simulink model "WSC_2023_Final_PVArray_Diode_All_Strings"  (R2023a)
settings: Solver=VariableStepAuto  StartTime=0.0  StopTime=1  FixedStep=Ts_Power  MinStep=0.0025  RelTol=1e-4
PreLoadFcn:
  | Ts_Power=5e-4;
  | Slope_Vdc=1;
InitFcn:
  | Ts_Power=50e-6;
  | Tc=1e-5;%break algebraic loop time constant
StopFcn:
  | if exist('I','var') && exist('V','var')
  |    figure(1)
  |    clf
  |    n=find(I>=0);
  |    n=n(end);
  |    Vglobal=V(1:n);
  |    Iglobal=I(1:n);
  | 
  | 
  |    Pglobal=Vglobal.*Iglobal;
  |    n=find(Pglobal==max(Pglobal));
  |    Pmax=Pglobal(n);
  |    Vmp=Vglobal(n);
  |    Imp=Iglobal(n);
  | 
  | 
  |    subplot(211)
  |    plot(Vglobal, Iglobal,Vmp,Imp,'or')
  |    ylabel('Current (A)')
  |    title(sprintf('Global I-V & P-V characteristics\n %s' ,ModuleName))
  | 
  | 
  |    subplot(212)
  |    plot(Vglobal, Pglobal,Vmp,Pmax,'or')
  |    ylabel('Power (W)')
  |    xlabel('Voltage (V)')
  | end
model workspace (MAT data in the model file):
  slope_Vdc = 3.0848387096
undefined symbols (not defined in the file or in its folder): Slope_Vdc_string1, Slope_Vdc_string2, Slope_Vdc_string3
libraries: spsPVArrayLib x257, spsVariableResistorLib x257, spsDiodeLib x55, spsCurrentMeasurementLib x3, spsVoltageMeasurementLib x3, spsControlledVoltageSourceLib x3, simulink x3, spspowerguiLib x3
(part 10 of 13)

== system WSC_2023_Final_PVArray_Diode_All_Strings/Subsystem22/PV7 ==
  Irr : Inport
  1PΩ : Constant  Value=1e15
  PV2 : spsPVArrayLib/PV Array  Npar=1  Nser=1  PlotType=array @ 25 deg.C & specified irradiances  S_vec="[ 1000  500  100 ]"  Temp_C_vec="[ 45 25  ]"  ModuleName=User-defined  PlotWhenSelected=off  Pm=3.8061  Ncell=1  Voc=0.7315  Isc=6.41  Vm=0.626  Im=6.08  beta_Voc_pc=-0.2256195755  alpha_Isc_pc=0.04692556634  beta_Voc=-0.0016504  alpha_Isc=0.0030079  IL=6.4137  I0=6.5578e-13  nI=0.95237  Rsh=7.312  Rs=0.0042689  RobustModel=on  RobustCellTemperature=25  BAL=on  Tc=1e-5  Tfilter=5e-5
  Terminator1 : Terminator
  Variable Resistor2 : spsVariableResistorLib/Variable Resistor  Rabsmin=1e-3
      settings: LibrarySourceBlock=sps_lib/Passives/Variable Resistor
  + : PMIOPort  Side=Left
  - : PMIOPort  Port=2  Side=Right
  wires:
  Irr/1 -> PV2/1
  1PΩ/1 -> Variable Resistor2/1
  PV2/1 -> Terminator1/1
  connections:
  -/RConn1 -- Variable Resistor2/RConn1 -- PV2/RConn2
  +/RConn1 -- Variable Resistor2/LConn1 -- PV2/RConn1

== system WSC_2023_Final_PVArray_Diode_All_Strings/Subsystem23/PV1 ==
  Irr : Inport
  1PΩ : Constant  Value=1e15
  PV2 : spsPVArrayLib/PV Array  Npar=1  Nser=1  PlotType=array @ 25 deg.C & specified irradiances  S_vec="[ 1000  500  100 ]"  Temp_C_vec="[ 45 25  ]"  ModuleName=User-defined  PlotWhenSelected=off  Pm=3.8061  Ncell=1  Voc=0.7315  Isc=6.41  Vm=0.626  Im=6.08  beta_Voc_pc=-0.2256195755  alpha_Isc_pc=0.04692556634  beta_Voc=-0.0016504  alpha_Isc=0.0030079  IL=6.4137  I0=6.5578e-13  nI=0.95237  Rsh=7.312  Rs=0.0042689  RobustModel=on  RobustCellTemperature=25  BAL=on  Tc=1e-5  Tfilter=5e-5
  Terminator1 : Terminator
  Variable Resistor2 : spsVariableResistorLib/Variable Resistor  Rabsmin=1e-3
      settings: LibrarySourceBlock=sps_lib/Passives/Variable Resistor
  + : PMIOPort  Side=Left
  - : PMIOPort  Port=2  Side=Right
  wires:
  Irr/1 -> PV2/1
  1PΩ/1 -> Variable Resistor2/1
  PV2/1 -> Terminator1/1
  connections:
  -/RConn1 -- Variable Resistor2/RConn1 -- PV2/RConn2
  +/RConn1 -- Variable Resistor2/LConn1 -- PV2/RConn1

== system WSC_2023_Final_PVArray_Diode_All_Strings/Subsystem23/PV2 ==
  Irr : Inport
  1PΩ : Constant  Value=1e15
  PV2 : spsPVArrayLib/PV Array  Npar=1  Nser=1  PlotType=array @ 25 deg.C & specified irradiances  S_vec="[ 1000  500  100 ]"  Temp_C_vec="[ 45 25  ]"  ModuleName=User-defined  PlotWhenSelected=off  Pm=3.8061  Ncell=1  Voc=0.7315  Isc=6.41  Vm=0.626  Im=6.08  beta_Voc_pc=-0.2256195755  alpha_Isc_pc=0.04692556634  beta_Voc=-0.0016504  alpha_Isc=0.0030079  IL=6.4137  I0=6.5578e-13  nI=0.95237  Rsh=7.312  Rs=0.0042689  RobustModel=on  RobustCellTemperature=25  BAL=on  Tc=1e-5  Tfilter=5e-5
  Terminator1 : Terminator
  Variable Resistor2 : spsVariableResistorLib/Variable Resistor  Rabsmin=1e-3
      settings: LibrarySourceBlock=sps_lib/Passives/Variable Resistor
  + : PMIOPort  Side=Left
  - : PMIOPort  Port=2  Side=Right
  wires:
  Irr/1 -> PV2/1
  1PΩ/1 -> Variable Resistor2/1
  PV2/1 -> Terminator1/1
  connections:
  -/RConn1 -- Variable Resistor2/RConn1 -- PV2/RConn2
  +/RConn1 -- Variable Resistor2/LConn1 -- PV2/RConn1

== system WSC_2023_Final_PVArray_Diode_All_Strings/Subsystem23/PV3 ==
  Irr : Inport
  1PΩ : Constant  Value=1e15
  PV2 : spsPVArrayLib/PV Array  Npar=1  Nser=1  PlotType=array @ 25 deg.C & specified irradiances  S_vec="[ 1000  500  100 ]"  Temp_C_vec="[ 45 25  ]"  ModuleName=User-defined  PlotWhenSelected=off  Pm=3.8061  Ncell=1  Voc=0.7315  Isc=6.41  Vm=0.626  Im=6.08  beta_Voc_pc=-0.2256195755  alpha_Isc_pc=0.04692556634  beta_Voc=-0.0016504  alpha_Isc=0.0030079  IL=6.4137  I0=6.5578e-13  nI=0.95237  Rsh=7.312  Rs=0.0042689  RobustModel=on  RobustCellTemperature=25  BAL=on  Tc=1e-5  Tfilter=5e-5
  Terminator1 : Terminator
  Variable Resistor2 : spsVariableResistorLib/Variable Resistor  Rabsmin=1e-3
      settings: LibrarySourceBlock=sps_lib/Passives/Variable Resistor
  + : PMIOPort  Side=Left
  - : PMIOPort  Port=2  Side=Right
  wires:
  Irr/1 -> PV2/1
  1PΩ/1 -> Variable Resistor2/1
  PV2/1 -> Terminator1/1
  connections:
  -/RConn1 -- Variable Resistor2/RConn1 -- PV2/RConn2
  +/RConn1 -- Variable Resistor2/LConn1 -- PV2/RConn1

== system WSC_2023_Final_PVArray_Diode_All_Strings/Subsystem23/PV4 ==
  Irr : Inport
  1PΩ : Constant  Value=1e15
  PV2 : spsPVArrayLib/PV Array  Npar=1  Nser=1  PlotType=array @ 25 deg.C & specified irradiances  S_vec="[ 1000  500  100 ]"  Temp_C_vec="[ 45 25  ]"  ModuleName=User-defined  PlotWhenSelected=off  Pm=3.8061  Ncell=1  Voc=0.7315  Isc=6.41  Vm=0.626  Im=6.08  beta_Voc_pc=-0.2256195755  alpha_Isc_pc=0.04692556634  beta_Voc=-0.0016504  alpha_Isc=0.0030079  IL=6.4137  I0=6.5578e-13  nI=0.95237  Rsh=7.312  Rs=0.0042689  RobustModel=on  RobustCellTemperature=25  BAL=on  Tc=1e-5  Tfilter=5e-5
  Terminator1 : Terminator
  Variable Resistor2 : spsVariableResistorLib/Variable Resistor  Rabsmin=1e-3
      settings: LibrarySourceBlock=sps_lib/Passives/Variable Resistor
  + : PMIOPort  Side=Left
  - : PMIOPort  Port=2  Side=Right
  wires:
  Irr/1 -> PV2/1
  1PΩ/1 -> Variable Resistor2/1
  PV2/1 -> Terminator1/1
  connections:
  -/RConn1 -- Variable Resistor2/RConn1 -- PV2/RConn2
  +/RConn1 -- Variable Resistor2/LConn1 -- PV2/RConn1

== system WSC_2023_Final_PVArray_Diode_All_Strings/Subsystem23/PV5 ==
  Irr : Inport
  1PΩ : Constant  Value=1e15
  PV2 : spsPVArrayLib/PV Array  Npar=1  Nser=1  PlotType=array @ 25 deg.C & specified irradiances  S_vec="[ 1000  500  100 ]"  Temp_C_vec="[ 45 25  ]"  ModuleName=User-defined  PlotWhenSelected=off  Pm=3.8061  Ncell=1  Voc=0.7315  Isc=6.41  Vm=0.626  Im=6.08  beta_Voc_pc=-0.2256195755  alpha_Isc_pc=0.04692556634  beta_Voc=-0.0016504  alpha_Isc=0.0030079  IL=6.4137  I0=6.5578e-13  nI=0.95237  Rsh=7.312  Rs=0.0042689  RobustModel=on  RobustCellTemperature=25  BAL=on  Tc=1e-5  Tfilter=5e-5
  Terminator1 : Terminator
  Variable Resistor2 : spsVariableResistorLib/Variable Resistor  Rabsmin=1e-3
      settings: LibrarySourceBlock=sps_lib/Passives/Variable Resistor
  + : PMIOPort  Side=Left
  - : PMIOPort  Port=2  Side=Right
  wires:
  Irr/1 -> PV2/1
  1PΩ/1 -> Variable Resistor2/1
  PV2/1 -> Terminator1/1
  connections:
  -/RConn1 -- Variable Resistor2/RConn1 -- PV2/RConn2
  +/RConn1 -- Variable Resistor2/LConn1 -- PV2/RConn1

== system WSC_2023_Final_PVArray_Diode_All_Strings/Subsystem23/PV6 ==
  Irr : Inport
  1PΩ : Constant  Value=1e15
  PV2 : spsPVArrayLib/PV Array  Npar=1  Nser=1  PlotType=array @ 25 deg.C & specified irradiances  S_vec="[ 1000  500  100 ]"  Temp_C_vec="[ 45 25  ]"  ModuleName=User-defined  PlotWhenSelected=off  Pm=3.8061  Ncell=1  Voc=0.7315  Isc=6.41  Vm=0.626  Im=6.08  beta_Voc_pc=-0.2256195755  alpha_Isc_pc=0.04692556634  beta_Voc=-0.0016504  alpha_Isc=0.0030079  IL=6.4137  I0=6.5578e-13  nI=0.95237  Rsh=7.312  Rs=0.0042689  RobustModel=on  RobustCellTemperature=25  BAL=on  Tc=1e-5  Tfilter=5e-5
  Terminator1 : Terminator
  Variable Resistor2 : spsVariableResistorLib/Variable Resistor  Rabsmin=1e-3
      settings: LibrarySourceBlock=sps_lib/Passives/Variable Resistor
  + : PMIOPort  Side=Left
  - : PMIOPort  Port=2  Side=Right
  wires:
  Irr/1 -> PV2/1
  1PΩ/1 -> Variable Resistor2/1
  PV2/1 -> Terminator1/1
  connections:
  -/RConn1 -- Variable Resistor2/RConn1 -- PV2/RConn2
  +/RConn1 -- Variable Resistor2/LConn1 -- PV2/RConn1

== system WSC_2023_Final_PVArray_Diode_All_Strings/Subsystem23/PV7 ==
  Irr : Inport
  1PΩ : Constant  Value=1e15
  PV2 : spsPVArrayLib/PV Array  Npar=1  Nser=1  PlotType=array @ 25 deg.C & specified irradiances  S_vec="[ 1000  500  100 ]"  Temp_C_vec="[ 45 25  ]"  ModuleName=User-defined  PlotWhenSelected=off  Pm=3.8061  Ncell=1  Voc=0.7315  Isc=6.41  Vm=0.626  Im=6.08  beta_Voc_pc=-0.2256195755  alpha_Isc_pc=0.04692556634  beta_Voc=-0.0016504  alpha_Isc=0.0030079  IL=6.4137  I0=6.5578e-13  nI=0.95237  Rsh=7.312  Rs=0.0042689  RobustModel=on  RobustCellTemperature=25  BAL=on  Tc=1e-5  Tfilter=5e-5
  Terminator1 : Terminator
  Variable Resistor2 : spsVariableResistorLib/Variable Resistor  Rabsmin=1e-3
      settings: LibrarySourceBlock=sps_lib/Passives/Variable Resistor
  + : PMIOPort  Side=Left
  - : PMIOPort  Port=2  Side=Right
  wires:
  Irr/1 -> PV2/1
  1PΩ/1 -> Variable Resistor2/1
  PV2/1 -> Terminator1/1
  connections:
  -/RConn1 -- Variable Resistor2/RConn1 -- PV2/RConn2
  +/RConn1 -- Variable Resistor2/LConn1 -- PV2/RConn1

== system WSC_2023_Final_PVArray_Diode_All_Strings/Subsystem24/PV1 ==
  Irr : Inport
  1PΩ : Constant  Value=1e15
  PV2 : spsPVArrayLib/PV Array  Npar=1  Nser=1  PlotType=array @ 25 deg.C & specified irradiances  S_vec="[ 1000  500  100 ]"  Temp_C_vec="[ 45 25  ]"  ModuleName=User-defined  PlotWhenSelected=off  Pm=3.8061  Ncell=1  Voc=0.7315  Isc=6.41  Vm=0.626  Im=6.08  beta_Voc_pc=-0.2256195755  alpha_Isc_pc=0.04692556634  beta_Voc=-0.0016504  alpha_Isc=0.0030079  IL=6.4137  I0=6.5578e-13  nI=0.95237  Rsh=7.312  Rs=0.0042689  RobustModel=on  RobustCellTemperature=25  BAL=on  Tc=1e-5  Tfilter=5e-5
  Terminator1 : Terminator
  Variable Resistor2 : spsVariableResistorLib/Variable Resistor  Rabsmin=1e-3
      settings: LibrarySourceBlock=sps_lib/Passives/Variable Resistor
  + : PMIOPort  Side=Left
  - : PMIOPort  Port=2  Side=Right
  wires:
  Irr/1 -> PV2/1
  1PΩ/1 -> Variable Resistor2/1
  PV2/1 -> Terminator1/1
  connections:
  -/RConn1 -- Variable Resistor2/RConn1 -- PV2/RConn2
  +/RConn1 -- Variable Resistor2/LConn1 -- PV2/RConn1

== system WSC_2023_Final_PVArray_Diode_All_Strings/Subsystem24/PV2 ==
  Irr : Inport
  1PΩ : Constant  Value=1e15
  PV2 : spsPVArrayLib/PV Array  Npar=1  Nser=1  PlotType=array @ 25 deg.C & specified irradiances  S_vec="[ 1000  500  100 ]"  Temp_C_vec="[ 45 25  ]"  ModuleName=User-defined  PlotWhenSelected=off  Pm=3.8061  Ncell=1  Voc=0.7315  Isc=6.41  Vm=0.626  Im=6.08  beta_Voc_pc=-0.2256195755  alpha_Isc_pc=0.04692556634  beta_Voc=-0.0016504  alpha_Isc=0.0030079  IL=6.4137  I0=6.5578e-13  nI=0.95237  Rsh=7.312  Rs=0.0042689  RobustModel=on  RobustCellTemperature=25  BAL=on  Tc=1e-5  Tfilter=5e-5
  Terminator1 : Terminator
  Variable Resistor2 : spsVariableResistorLib/Variable Resistor  Rabsmin=1e-3
      settings: LibrarySourceBlock=sps_lib/Passives/Variable Resistor
  + : PMIOPort  Side=Left
  - : PMIOPort  Port=2  Side=Right
  wires:
  Irr/1 -> PV2/1
  1PΩ/1 -> Variable Resistor2/1
  PV2/1 -> Terminator1/1
  connections:
  -/RConn1 -- Variable Resistor2/RConn1 -- PV2/RConn2
  +/RConn1 -- Variable Resistor2/LConn1 -- PV2/RConn1

== system WSC_2023_Final_PVArray_Diode_All_Strings/Subsystem24/PV3 ==
  Irr : Inport
  1PΩ : Constant  Value=1e15
  PV2 : spsPVArrayLib/PV Array  Npar=1  Nser=1  PlotType=array @ 25 deg.C & specified irradiances  S_vec="[ 1000  500  100 ]"  Temp_C_vec="[ 45 25  ]"  ModuleName=User-defined  PlotWhenSelected=off  Pm=3.8061  Ncell=1  Voc=0.7315  Isc=6.41  Vm=0.626  Im=6.08  beta_Voc_pc=-0.2256195755  alpha_Isc_pc=0.04692556634  beta_Voc=-0.0016504  alpha_Isc=0.0030079  IL=6.4137  I0=6.5578e-13  nI=0.95237  Rsh=7.312  Rs=0.0042689  RobustModel=on  RobustCellTemperature=25  BAL=on  Tc=1e-5  Tfilter=5e-5
  Terminator1 : Terminator
  Variable Resistor2 : spsVariableResistorLib/Variable Resistor  Rabsmin=1e-3
      settings: LibrarySourceBlock=sps_lib/Passives/Variable Resistor
  + : PMIOPort  Side=Left
  - : PMIOPort  Port=2  Side=Right
  wires:
  Irr/1 -> PV2/1
  1PΩ/1 -> Variable Resistor2/1
  PV2/1 -> Terminator1/1
  connections:
  -/RConn1 -- Variable Resistor2/RConn1 -- PV2/RConn2
  +/RConn1 -- Variable Resistor2/LConn1 -- PV2/RConn1

== system WSC_2023_Final_PVArray_Diode_All_Strings/Subsystem24/PV4 ==
  Irr : Inport
  1PΩ : Constant  Value=1e15
  PV2 : spsPVArrayLib/PV Array  Npar=1  Nser=1  PlotType=array @ 25 deg.C & specified irradiances  S_vec="[ 1000  500  100 ]"  Temp_C_vec="[ 45 25  ]"  ModuleName=User-defined  PlotWhenSelected=off  Pm=3.8061  Ncell=1  Voc=0.7315  Isc=6.41  Vm=0.626  Im=6.08  beta_Voc_pc=-0.2256195755  alpha_Isc_pc=0.04692556634  beta_Voc=-0.0016504  alpha_Isc=0.0030079  IL=6.4137  I0=6.5578e-13  nI=0.95237  Rsh=7.312  Rs=0.0042689  RobustModel=on  RobustCellTemperature=25  BAL=on  Tc=1e-5  Tfilter=5e-5
  Terminator1 : Terminator
  Variable Resistor2 : spsVariableResistorLib/Variable Resistor  Rabsmin=1e-3
      settings: LibrarySourceBlock=sps_lib/Passives/Variable Resistor
  + : PMIOPort  Side=Left
  - : PMIOPort  Port=2  Side=Right
  wires:
  Irr/1 -> PV2/1
  1PΩ/1 -> Variable Resistor2/1
  PV2/1 -> Terminator1/1
  connections:
  -/RConn1 -- Variable Resistor2/RConn1 -- PV2/RConn2
  +/RConn1 -- Variable Resistor2/LConn1 -- PV2/RConn1

== system WSC_2023_Final_PVArray_Diode_All_Strings/Subsystem24/PV5 ==
  Irr : Inport
  1PΩ : Constant  Value=1e15
  PV2 : spsPVArrayLib/PV Array  Npar=1  Nser=1  PlotType=array @ 25 deg.C & specified irradiances  S_vec="[ 1000  500  100 ]"  Temp_C_vec="[ 45 25  ]"  ModuleName=User-defined  PlotWhenSelected=off  Pm=3.8061  Ncell=1  Voc=0.7315  Isc=6.41  Vm=0.626  Im=6.08  beta_Voc_pc=-0.2256195755  alpha_Isc_pc=0.04692556634  beta_Voc=-0.0016504  alpha_Isc=0.0030079  IL=6.4137  I0=6.5578e-13  nI=0.95237  Rsh=7.312  Rs=0.0042689  RobustModel=on  RobustCellTemperature=25  BAL=on  Tc=1e-5  Tfilter=5e-5
  Terminator1 : Terminator
  Variable Resistor2 : spsVariableResistorLib/Variable Resistor  Rabsmin=1e-3
      settings: LibrarySourceBlock=sps_lib/Passives/Variable Resistor
  + : PMIOPort  Side=Left
  - : PMIOPort  Port=2  Side=Right
  wires:
  Irr/1 -> PV2/1
  1PΩ/1 -> Variable Resistor2/1
  PV2/1 -> Terminator1/1
  connections:
  -/RConn1 -- Variable Resistor2/RConn1 -- PV2/RConn2
  +/RConn1 -- Variable Resistor2/LConn1 -- PV2/RConn1

== system WSC_2023_Final_PVArray_Diode_All_Strings/Subsystem24/PV6 ==
  Irr : Inport
  1PΩ : Constant  Value=1e15
  PV2 : spsPVArrayLib/PV Array  Npar=1  Nser=1  PlotType=array @ 25 deg.C & specified irradiances  S_vec="[ 1000  500  100 ]"  Temp_C_vec="[ 45 25  ]"  ModuleName=User-defined  PlotWhenSelected=off  Pm=3.8061  Ncell=1  Voc=0.7315  Isc=6.41  Vm=0.626  Im=6.08  beta_Voc_pc=-0.2256195755  alpha_Isc_pc=0.04692556634  beta_Voc=-0.0016504  alpha_Isc=0.0030079  IL=6.4137  I0=6.5578e-13  nI=0.95237  Rsh=7.312  Rs=0.0042689  RobustModel=on  RobustCellTemperature=25  BAL=on  Tc=1e-5  Tfilter=5e-5
  Terminator1 : Terminator
  Variable Resistor2 : spsVariableResistorLib/Variable Resistor  Rabsmin=1e-3
      settings: LibrarySourceBlock=sps_lib/Passives/Variable Resistor
  + : PMIOPort  Side=Left
  - : PMIOPort  Port=2  Side=Right
  wires:
  Irr/1 -> PV2/1
  1PΩ/1 -> Variable Resistor2/1
  PV2/1 -> Terminator1/1
  connections:
  -/RConn1 -- Variable Resistor2/RConn1 -- PV2/RConn2
  +/RConn1 -- Variable Resistor2/LConn1 -- PV2/RConn1

== system WSC_2023_Final_PVArray_Diode_All_Strings/Subsystem24/PV7 ==
  Irr : Inport
  1PΩ : Constant  Value=1e15
  PV2 : spsPVArrayLib/PV Array  Npar=1  Nser=1  PlotType=array @ 25 deg.C & specified irradiances  S_vec="[ 1000  500  100 ]"  Temp_C_vec="[ 45 25  ]"  ModuleName=User-defined  PlotWhenSelected=off  Pm=3.8061  Ncell=1  Voc=0.7315  Isc=6.41  Vm=0.626  Im=6.08  beta_Voc_pc=-0.2256195755  alpha_Isc_pc=0.04692556634  beta_Voc=-0.0016504  alpha_Isc=0.0030079  IL=6.4137  I0=6.5578e-13  nI=0.95237  Rsh=7.312  Rs=0.0042689  RobustModel=on  RobustCellTemperature=25  BAL=on  Tc=1e-5  Tfilter=5e-5
  Terminator1 : Terminator
  Variable Resistor2 : spsVariableResistorLib/Variable Resistor  Rabsmin=1e-3
      settings: LibrarySourceBlock=sps_lib/Passives/Variable Resistor
  + : PMIOPort  Side=Left
  - : PMIOPort  Port=2  Side=Right
  wires:
  Irr/1 -> PV2/1
  1PΩ/1 -> Variable Resistor2/1
  PV2/1 -> Terminator1/1
  connections:
  -/RConn1 -- Variable Resistor2/RConn1 -- PV2/RConn2
  +/RConn1 -- Variable Resistor2/LConn1 -- PV2/RConn1

== system WSC_2023_Final_PVArray_Diode_All_Strings/Subsystem26/PV1 ==
  Irr : Inport
  1PΩ : Constant  Value=1e15
  PV2 : spsPVArrayLib/PV Array  Npar=1  Nser=1  PlotType=array @ 25 deg.C & specified irradiances  S_vec="[ 1000  500  100 ]"  Temp_C_vec="[ 45 25  ]"  ModuleName=User-defined  PlotWhenSelected=off  Pm=3.8061  Ncell=1  Voc=0.7315  Isc=6.41  Vm=0.626  Im=6.08  beta_Voc_pc=-0.2256195755  alpha_Isc_pc=0.04692556634  beta_Voc=-0.0016504  alpha_Isc=0.0030079  IL=6.4137  I0=6.5578e-13  nI=0.95237  Rsh=7.312  Rs=0.0042689  RobustModel=on  RobustCellTemperature=25  BAL=on  Tc=1e-5  Tfilter=5e-5
  Terminator1 : Terminator
  Variable Resistor2 : spsVariableResistorLib/Variable Resistor  Rabsmin=1e-3
      settings: LibrarySourceBlock=sps_lib/Passives/Variable Resistor
  + : PMIOPort  Side=Left
  - : PMIOPort  Port=2  Side=Right
  wires:
  Irr/1 -> PV2/1
  1PΩ/1 -> Variable Resistor2/1
  PV2/1 -> Terminator1/1
  connections:
  -/RConn1 -- Variable Resistor2/RConn1 -- PV2/RConn2
  +/RConn1 -- Variable Resistor2/LConn1 -- PV2/RConn1

== system WSC_2023_Final_PVArray_Diode_All_Strings/Subsystem26/PV2 ==
  Irr : Inport
  1PΩ : Constant  Value=1e15
  PV2 : spsPVArrayLib/PV Array  Npar=1  Nser=1  PlotType=array @ 25 deg.C & specified irradiances  S_vec="[ 1000  500  100 ]"  Temp_C_vec="[ 45 25  ]"  ModuleName=User-defined  PlotWhenSelected=off  Pm=3.8061  Ncell=1  Voc=0.7315  Isc=6.41  Vm=0.626  Im=6.08  beta_Voc_pc=-0.2256195755  alpha_Isc_pc=0.04692556634  beta_Voc=-0.0016504  alpha_Isc=0.0030079  IL=6.4137  I0=6.5578e-13  nI=0.95237  Rsh=7.312  Rs=0.0042689  RobustModel=on  RobustCellTemperature=25  BAL=on  Tc=1e-5  Tfilter=5e-5
  Terminator1 : Terminator
  Variable Resistor2 : spsVariableResistorLib/Variable Resistor  Rabsmin=1e-3
      settings: LibrarySourceBlock=sps_lib/Passives/Variable Resistor
  + : PMIOPort  Side=Left
  - : PMIOPort  Port=2  Side=Right
  wires:
  Irr/1 -> PV2/1
  1PΩ/1 -> Variable Resistor2/1
  PV2/1 -> Terminator1/1
  connections:
  -/RConn1 -- Variable Resistor2/RConn1 -- PV2/RConn2
  +/RConn1 -- Variable Resistor2/LConn1 -- PV2/RConn1

== system WSC_2023_Final_PVArray_Diode_All_Strings/Subsystem26/PV3 ==
  Irr : Inport
  1PΩ : Constant  Value=1e15
  PV2 : spsPVArrayLib/PV Array  Npar=1  Nser=1  PlotType=array @ 25 deg.C & specified irradiances  S_vec="[ 1000  500  100 ]"  Temp_C_vec="[ 45 25  ]"  ModuleName=User-defined  PlotWhenSelected=off  Pm=3.8061  Ncell=1  Voc=0.7315  Isc=6.41  Vm=0.626  Im=6.08  beta_Voc_pc=-0.2256195755  alpha_Isc_pc=0.04692556634  beta_Voc=-0.0016504  alpha_Isc=0.0030079  IL=6.4137  I0=6.5578e-13  nI=0.95237  Rsh=7.312  Rs=0.0042689  RobustModel=on  RobustCellTemperature=25  BAL=on  Tc=1e-5  Tfilter=5e-5
  Terminator1 : Terminator
  Variable Resistor2 : spsVariableResistorLib/Variable Resistor  Rabsmin=1e-3
      settings: LibrarySourceBlock=sps_lib/Passives/Variable Resistor
  + : PMIOPort  Side=Left
  - : PMIOPort  Port=2  Side=Right
  wires:
  Irr/1 -> PV2/1
  1PΩ/1 -> Variable Resistor2/1
  PV2/1 -> Terminator1/1
  connections:
  -/RConn1 -- Variable Resistor2/RConn1 -- PV2/RConn2
  +/RConn1 -- Variable Resistor2/LConn1 -- PV2/RConn1

== system WSC_2023_Final_PVArray_Diode_All_Strings/Subsystem26/PV4 ==
  Irr : Inport
  1PΩ : Constant  Value=1e15
  PV2 : spsPVArrayLib/PV Array  Npar=1  Nser=1  PlotType=array @ 25 deg.C & specified irradiances  S_vec="[ 1000  500  100 ]"  Temp_C_vec="[ 45 25  ]"  ModuleName=User-defined  PlotWhenSelected=off  Pm=3.8061  Ncell=1  Voc=0.7315  Isc=6.41  Vm=0.626  Im=6.08  beta_Voc_pc=-0.2256195755  alpha_Isc_pc=0.04692556634  beta_Voc=-0.0016504  alpha_Isc=0.0030079  IL=6.4137  I0=6.5578e-13  nI=0.95237  Rsh=7.312  Rs=0.0042689  RobustModel=on  RobustCellTemperature=25  BAL=on  Tc=1e-5  Tfilter=5e-5
  Terminator1 : Terminator
  Variable Resistor2 : spsVariableResistorLib/Variable Resistor  Rabsmin=1e-3
      settings: LibrarySourceBlock=sps_lib/Passives/Variable Resistor
  + : PMIOPort  Side=Left
  - : PMIOPort  Port=2  Side=Right
  wires:
  Irr/1 -> PV2/1
  1PΩ/1 -> Variable Resistor2/1
  PV2/1 -> Terminator1/1
  connections:
  -/RConn1 -- Variable Resistor2/RConn1 -- PV2/RConn2
  +/RConn1 -- Variable Resistor2/LConn1 -- PV2/RConn1

== system WSC_2023_Final_PVArray_Diode_All_Strings/Subsystem26/PV5 ==
  Irr : Inport
  1PΩ : Constant  Value=1e15
  PV2 : spsPVArrayLib/PV Array  Npar=1  Nser=1  PlotType=array @ 25 deg.C & specified irradiances  S_vec="[ 1000  500  100 ]"  Temp_C_vec="[ 45 25  ]"  ModuleName=User-defined  PlotWhenSelected=off  Pm=3.8061  Ncell=1  Voc=0.7315  Isc=6.41  Vm=0.626  Im=6.08  beta_Voc_pc=-0.2256195755  alpha_Isc_pc=0.04692556634  beta_Voc=-0.0016504  alpha_Isc=0.0030079  IL=6.4137  I0=6.5578e-13  nI=0.95237  Rsh=7.312  Rs=0.0042689  RobustModel=on  RobustCellTemperature=25  BAL=on  Tc=1e-5  Tfilter=5e-5
  Terminator1 : Terminator
  Variable Resistor2 : spsVariableResistorLib/Variable Resistor  Rabsmin=1e-3
      settings: LibrarySourceBlock=sps_lib/Passives/Variable Resistor
  + : PMIOPort  Side=Left
  - : PMIOPort  Port=2  Side=Right
  wires:
  Irr/1 -> PV2/1
  1PΩ/1 -> Variable Resistor2/1
  PV2/1 -> Terminator1/1
  connections:
  -/RConn1 -- Variable Resistor2/RConn1 -- PV2/RConn2
  +/RConn1 -- Variable Resistor2/LConn1 -- PV2/RConn1

== system WSC_2023_Final_PVArray_Diode_All_Strings/Subsystem26/PV6 ==
  Irr : Inport
  1PΩ : Constant  Value=1e15
  PV2 : spsPVArrayLib/PV Array  Npar=1  Nser=1  PlotType=array @ 25 deg.C & specified irradiances  S_vec="[ 1000  500  100 ]"  Temp_C_vec="[ 45 25  ]"  ModuleName=User-defined  PlotWhenSelected=off  Pm=3.8061  Ncell=1  Voc=0.7315  Isc=6.41  Vm=0.626  Im=6.08  beta_Voc_pc=-0.2256195755  alpha_Isc_pc=0.04692556634  beta_Voc=-0.0016504  alpha_Isc=0.0030079  IL=6.4137  I0=6.5578e-13  nI=0.95237  Rsh=7.312  Rs=0.0042689  RobustModel=on  RobustCellTemperature=25  BAL=on  Tc=1e-5  Tfilter=5e-5
  Terminator1 : Terminator
  Variable Resistor2 : spsVariableResistorLib/Variable Resistor  Rabsmin=1e-3
      settings: LibrarySourceBlock=sps_lib/Passives/Variable Resistor
  + : PMIOPort  Side=Left
  - : PMIOPort  Port=2  Side=Right
  wires:
  Irr/1 -> PV2/1
  1PΩ/1 -> Variable Resistor2/1
  PV2/1 -> Terminator1/1
  connections:
  -/RConn1 -- Variable Resistor2/RConn1 -- PV2/RConn2
  +/RConn1 -- Variable Resistor2/LConn1 -- PV2/RConn1

== system WSC_2023_Final_PVArray_Diode_All_Strings/Subsystem27/PV1 ==
  Irr : Inport
  1PΩ : Constant  Value=1e15
  PV2 : spsPVArrayLib/PV Array  Npar=1  Nser=1  PlotType=array @ 25 deg.C & specified irradiances  S_vec="[ 1000  500  100 ]"  Temp_C_vec="[ 45 25  ]"  ModuleName=User-defined  PlotWhenSelected=off  Pm=3.8061  Ncell=1  Voc=0.7315  Isc=6.41  Vm=0.626  Im=6.08  beta_Voc_pc=-0.2256195755  alpha_Isc_pc=0.04692556634  beta_Voc=-0.0016504  alpha_Isc=0.0030079  IL=6.4137  I0=6.5578e-13  nI=0.95237  Rsh=7.312  Rs=0.0042689  RobustModel=on  RobustCellTemperature=25  BAL=on  Tc=1e-5  Tfilter=5e-5
  Terminator1 : Terminator
  Variable Resistor2 : spsVariableResistorLib/Variable Resistor  Rabsmin=1e-3
      settings: LibrarySourceBlock=sps_lib/Passives/Variable Resistor
  + : PMIOPort  Side=Left
  - : PMIOPort  Port=2  Side=Right
  wires:
  Irr/1 -> PV2/1
  1PΩ/1 -> Variable Resistor2/1
  PV2/1 -> Terminator1/1
  connections:
  -/RConn1 -- Variable Resistor2/RConn1 -- PV2/RConn2
  +/RConn1 -- Variable Resistor2/LConn1 -- PV2/RConn1

== system WSC_2023_Final_PVArray_Diode_All_Strings/Subsystem27/PV2 ==
  Irr : Inport
  1PΩ : Constant  Value=1e15
  PV2 : spsPVArrayLib/PV Array  Npar=1  Nser=1  PlotType=array @ 25 deg.C & specified irradiances  S_vec="[ 1000  500  100 ]"  Temp_C_vec="[ 45 25  ]"  ModuleName=User-defined  PlotWhenSelected=off  Pm=3.8061  Ncell=1  Voc=0.7315  Isc=6.41  Vm=0.626  Im=6.08  beta_Voc_pc=-0.2256195755  alpha_Isc_pc=0.04692556634  beta_Voc=-0.0016504  alpha_Isc=0.0030079  IL=6.4137  I0=6.5578e-13  nI=0.95237  Rsh=7.312  Rs=0.0042689  RobustModel=on  RobustCellTemperature=25  BAL=on  Tc=1e-5  Tfilter=5e-5
  Terminator1 : Terminator
  Variable Resistor2 : spsVariableResistorLib/Variable Resistor  Rabsmin=1e-3
      settings: LibrarySourceBlock=sps_lib/Passives/Variable Resistor
  + : PMIOPort  Side=Left
  - : PMIOPort  Port=2  Side=Right
  wires:
  Irr/1 -> PV2/1
  1PΩ/1 -> Variable Resistor2/1
  PV2/1 -> Terminator1/1
  connections:
  -/RConn1 -- Variable Resistor2/RConn1 -- PV2/RConn2
  +/RConn1 -- Variable Resistor2/LConn1 -- PV2/RConn1

== system WSC_2023_Final_PVArray_Diode_All_Strings/Subsystem27/PV3 ==
  Irr : Inport
  1PΩ : Constant  Value=1e15
  PV2 : spsPVArrayLib/PV Array  Npar=1  Nser=1  PlotType=array @ 25 deg.C & specified irradiances  S_vec="[ 1000  500  100 ]"  Temp_C_vec="[ 45 25  ]"  ModuleName=User-defined  PlotWhenSelected=off  Pm=3.8061  Ncell=1  Voc=0.7315  Isc=6.41  Vm=0.626  Im=6.08  beta_Voc_pc=-0.2256195755  alpha_Isc_pc=0.04692556634  beta_Voc=-0.0016504  alpha_Isc=0.0030079  IL=6.4137  I0=6.5578e-13  nI=0.95237  Rsh=7.312  Rs=0.0042689  RobustModel=on  RobustCellTemperature=25  BAL=on  Tc=1e-5  Tfilter=5e-5
  Terminator1 : Terminator
  Variable Resistor2 : spsVariableResistorLib/Variable Resistor  Rabsmin=1e-3
      settings: LibrarySourceBlock=sps_lib/Passives/Variable Resistor
  + : PMIOPort  Side=Left
  - : PMIOPort  Port=2  Side=Right
  wires:
  Irr/1 -> PV2/1
  1PΩ/1 -> Variable Resistor2/1
  PV2/1 -> Terminator1/1
  connections:
  -/RConn1 -- Variable Resistor2/RConn1 -- PV2/RConn2
  +/RConn1 -- Variable Resistor2/LConn1 -- PV2/RConn1

== system WSC_2023_Final_PVArray_Diode_All_Strings/Subsystem27/PV4 ==
  Irr : Inport
  1PΩ : Constant  Value=1e15
  PV2 : spsPVArrayLib/PV Array  Npar=1  Nser=1  PlotType=array @ 25 deg.C & specified irradiances  S_vec="[ 1000  500  100 ]"  Temp_C_vec="[ 45 25  ]"  ModuleName=User-defined  PlotWhenSelected=off  Pm=3.8061  Ncell=1  Voc=0.7315  Isc=6.41  Vm=0.626  Im=6.08  beta_Voc_pc=-0.2256195755  alpha_Isc_pc=0.04692556634  beta_Voc=-0.0016504  alpha_Isc=0.0030079  IL=6.4137  I0=6.5578e-13  nI=0.95237  Rsh=7.312  Rs=0.0042689  RobustModel=on  RobustCellTemperature=25  BAL=on  Tc=1e-5  Tfilter=5e-5
  Terminator1 : Terminator
  Variable Resistor2 : spsVariableResistorLib/Variable Resistor  Rabsmin=1e-3
      settings: LibrarySourceBlock=sps_lib/Passives/Variable Resistor
  + : PMIOPort  Side=Left
  - : PMIOPort  Port=2  Side=Right
  wires:
  Irr/1 -> PV2/1
  1PΩ/1 -> Variable Resistor2/1
  PV2/1 -> Terminator1/1
  connections:
  -/RConn1 -- Variable Resistor2/RConn1 -- PV2/RConn2
  +/RConn1 -- Variable Resistor2/LConn1 -- PV2/RConn1

== system WSC_2023_Final_PVArray_Diode_All_Strings/Subsystem27/PV5 ==
  Irr : Inport
  1PΩ : Constant  Value=1e15
  PV2 : spsPVArrayLib/PV Array  Npar=1  Nser=1  PlotType=array @ 25 deg.C & specified irradiances  S_vec="[ 1000  500  100 ]"  Temp_C_vec="[ 45 25  ]"  ModuleName=User-defined  PlotWhenSelected=off  Pm=3.8061  Ncell=1  Voc=0.7315  Isc=6.41  Vm=0.626  Im=6.08  beta_Voc_pc=-0.2256195755  alpha_Isc_pc=0.04692556634  beta_Voc=-0.0016504  alpha_Isc=0.0030079  IL=6.4137  I0=6.5578e-13  nI=0.95237  Rsh=7.312  Rs=0.0042689  RobustModel=on  RobustCellTemperature=25  BAL=on  Tc=1e-5  Tfilter=5e-5
  Terminator1 : Terminator
  Variable Resistor2 : spsVariableResistorLib/Variable Resistor  Rabsmin=1e-3
      settings: LibrarySourceBlock=sps_lib/Passives/Variable Resistor
  + : PMIOPort  Side=Left
  - : PMIOPort  Port=2  Side=Right
  wires:
  Irr/1 -> PV2/1
  1PΩ/1 -> Variable Resistor2/1
  PV2/1 -> Terminator1/1
  connections:
  -/RConn1 -- Variable Resistor2/RConn1 -- PV2/RConn2
  +/RConn1 -- Variable Resistor2/LConn1 -- PV2/RConn1

== system WSC_2023_Final_PVArray_Diode_All_Strings/Subsystem27/PV6 ==
  Irr : Inport
  1PΩ : Constant  Value=1e15
  PV2 : spsPVArrayLib/PV Array  Npar=1  Nser=1  PlotType=array @ 25 deg.C & specified irradiances  S_vec="[ 1000  500  100 ]"  Temp_C_vec="[ 45 25  ]"  ModuleName=User-defined  PlotWhenSelected=off  Pm=3.8061  Ncell=1  Voc=0.7315  Isc=6.41  Vm=0.626  Im=6.08  beta_Voc_pc=-0.2256195755  alpha_Isc_pc=0.04692556634  beta_Voc=-0.0016504  alpha_Isc=0.0030079  IL=6.4137  I0=6.5578e-13  nI=0.95237  Rsh=7.312  Rs=0.0042689  RobustModel=on  RobustCellTemperature=25  BAL=on  Tc=1e-5  Tfilter=5e-5
  Terminator1 : Terminator
  Variable Resistor2 : spsVariableResistorLib/Variable Resistor  Rabsmin=1e-3
      settings: LibrarySourceBlock=sps_lib/Passives/Variable Resistor
  + : PMIOPort  Side=Left
  - : PMIOPort  Port=2  Side=Right
  wires:
  Irr/1 -> PV2/1
  1PΩ/1 -> Variable Resistor2/1
  PV2/1 -> Terminator1/1
  connections:
  -/RConn1 -- Variable Resistor2/RConn1 -- PV2/RConn2
  +/RConn1 -- Variable Resistor2/LConn1 -- PV2/RConn1

== system WSC_2023_Final_PVArray_Diode_All_Strings/Subsystem28/PV1 ==
  Irr : Inport
  1PΩ : Constant  Value=1e15
  PV2 : spsPVArrayLib/PV Array  Npar=1  Nser=1  PlotType=array @ 25 deg.C & specified irradiances  S_vec="[ 1000  500  100 ]"  Temp_C_vec="[ 45 25  ]"  ModuleName=User-defined  PlotWhenSelected=off  Pm=3.8061  Ncell=1  Voc=0.7315  Isc=6.41  Vm=0.626  Im=6.08  beta_Voc_pc=-0.2256195755  alpha_Isc_pc=0.04692556634  beta_Voc=-0.0016504  alpha_Isc=0.0030079  IL=6.4137  I0=6.5578e-13  nI=0.95237  Rsh=7.312  Rs=0.0042689  RobustModel=on  RobustCellTemperature=25  BAL=on  Tc=1e-5  Tfilter=5e-5
  Terminator1 : Terminator
  Variable Resistor2 : spsVariableResistorLib/Variable Resistor  Rabsmin=1e-3
      settings: LibrarySourceBlock=sps_lib/Passives/Variable Resistor
  + : PMIOPort  Side=Left
  - : PMIOPort  Port=2  Side=Right
  wires:
  Irr/1 -> PV2/1
  1PΩ/1 -> Variable Resistor2/1
  PV2/1 -> Terminator1/1
  connections:
  -/RConn1 -- Variable Resistor2/RConn1 -- PV2/RConn2
  +/RConn1 -- Variable Resistor2/LConn1 -- PV2/RConn1

== system WSC_2023_Final_PVArray_Diode_All_Strings/Subsystem28/PV2 ==
  Irr : Inport
  1PΩ : Constant  Value=1e15
  PV2 : spsPVArrayLib/PV Array  Npar=1  Nser=1  PlotType=array @ 25 deg.C & specified irradiances  S_vec="[ 1000  500  100 ]"  Temp_C_vec="[ 45 25  ]"  ModuleName=User-defined  PlotWhenSelected=off  Pm=3.8061  Ncell=1  Voc=0.7315  Isc=6.41  Vm=0.626  Im=6.08  beta_Voc_pc=-0.2256195755  alpha_Isc_pc=0.04692556634  beta_Voc=-0.0016504  alpha_Isc=0.0030079  IL=6.4137  I0=6.5578e-13  nI=0.95237  Rsh=7.312  Rs=0.0042689  RobustModel=on  RobustCellTemperature=25  BAL=on  Tc=1e-5  Tfilter=5e-5
  Terminator1 : Terminator
  Variable Resistor2 : spsVariableResistorLib/Variable Resistor  Rabsmin=1e-3
      settings: LibrarySourceBlock=sps_lib/Passives/Variable Resistor
  + : PMIOPort  Side=Left
  - : PMIOPort  Port=2  Side=Right
  wires:
  Irr/1 -> PV2/1
  1PΩ/1 -> Variable Resistor2/1
  PV2/1 -> Terminator1/1
  connections:
  -/RConn1 -- Variable Resistor2/RConn1 -- PV2/RConn2
  +/RConn1 -- Variable Resistor2/LConn1 -- PV2/RConn1

== system WSC_2023_Final_PVArray_Diode_All_Strings/Subsystem28/PV3 ==
  Irr : Inport
  1PΩ : Constant  Value=1e15
  PV2 : spsPVArrayLib/PV Array  Npar=1  Nser=1  PlotType=array @ 25 deg.C & specified irradiances  S_vec="[ 1000  500  100 ]"  Temp_C_vec="[ 45 25  ]"  ModuleName=User-defined  PlotWhenSelected=off  Pm=3.8061  Ncell=1  Voc=0.7315  Isc=6.41  Vm=0.626  Im=6.08  beta_Voc_pc=-0.2256195755  alpha_Isc_pc=0.04692556634  beta_Voc=-0.0016504  alpha_Isc=0.0030079  IL=6.4137  I0=6.5578e-13  nI=0.95237  Rsh=7.312  Rs=0.0042689  RobustModel=on  RobustCellTemperature=25  BAL=on  Tc=1e-5  Tfilter=5e-5
  Terminator1 : Terminator
  Variable Resistor2 : spsVariableResistorLib/Variable Resistor  Rabsmin=1e-3
      settings: LibrarySourceBlock=sps_lib/Passives/Variable Resistor
  + : PMIOPort  Side=Left
  - : PMIOPort  Port=2  Side=Right
  wires:
  Irr/1 -> PV2/1
  1PΩ/1 -> Variable Resistor2/1
  PV2/1 -> Terminator1/1
  connections:
  -/RConn1 -- Variable Resistor2/RConn1 -- PV2/RConn2
  +/RConn1 -- Variable Resistor2/LConn1 -- PV2/RConn1

== system WSC_2023_Final_PVArray_Diode_All_Strings/Subsystem28/PV4 ==
  Irr : Inport
  1PΩ : Constant  Value=1e15
  PV2 : spsPVArrayLib/PV Array  Npar=1  Nser=1  PlotType=array @ 25 deg.C & specified irradiances  S_vec="[ 1000  500  100 ]"  Temp_C_vec="[ 45 25  ]"  ModuleName=User-defined  PlotWhenSelected=off  Pm=3.8061  Ncell=1  Voc=0.7315  Isc=6.41  Vm=0.626  Im=6.08  beta_Voc_pc=-0.2256195755  alpha_Isc_pc=0.04692556634  beta_Voc=-0.0016504  alpha_Isc=0.0030079  IL=6.4137  I0=6.5578e-13  nI=0.95237  Rsh=7.312  Rs=0.0042689  RobustModel=on  RobustCellTemperature=25  BAL=on  Tc=1e-5  Tfilter=5e-5
  Terminator1 : Terminator
  Variable Resistor2 : spsVariableResistorLib/Variable Resistor  Rabsmin=1e-3
      settings: LibrarySourceBlock=sps_lib/Passives/Variable Resistor
  + : PMIOPort  Side=Left
  - : PMIOPort  Port=2  Side=Right
  wires:
  Irr/1 -> PV2/1
  1PΩ/1 -> Variable Resistor2/1
  PV2/1 -> Terminator1/1
  connections:
  -/RConn1 -- Variable Resistor2/RConn1 -- PV2/RConn2
  +/RConn1 -- Variable Resistor2/LConn1 -- PV2/RConn1

== system WSC_2023_Final_PVArray_Diode_All_Strings/Subsystem28/PV5 ==
  Irr : Inport
  1PΩ : Constant  Value=1e15
  PV2 : spsPVArrayLib/PV Array  Npar=1  Nser=1  PlotType=array @ 25 deg.C & specified irradiances  S_vec="[ 1000  500  100 ]"  Temp_C_vec="[ 45 25  ]"  ModuleName=User-defined  PlotWhenSelected=off  Pm=3.8061  Ncell=1  Voc=0.7315  Isc=6.41  Vm=0.626  Im=6.08  beta_Voc_pc=-0.2256195755  alpha_Isc_pc=0.04692556634  beta_Voc=-0.0016504  alpha_Isc=0.0030079  IL=6.4137  I0=6.5578e-13  nI=0.95237  Rsh=7.312  Rs=0.0042689  RobustModel=on  RobustCellTemperature=25  BAL=on  Tc=1e-5  Tfilter=5e-5
  Terminator1 : Terminator
  Variable Resistor2 : spsVariableResistorLib/Variable Resistor  Rabsmin=1e-3
      settings: LibrarySourceBlock=sps_lib/Passives/Variable Resistor
  + : PMIOPort  Side=Left
  - : PMIOPort  Port=2  Side=Right
  wires:
  Irr/1 -> PV2/1
  1PΩ/1 -> Variable Resistor2/1
  PV2/1 -> Terminator1/1
  connections:
  -/RConn1 -- Variable Resistor2/RConn1 -- PV2/RConn2
  +/RConn1 -- Variable Resistor2/LConn1 -- PV2/RConn1

== system WSC_2023_Final_PVArray_Diode_All_Strings/Subsystem28/PV6 ==
  Irr : Inport
  1PΩ : Constant  Value=1e15
  PV2 : spsPVArrayLib/PV Array  Npar=1  Nser=1  PlotType=array @ 25 deg.C & specified irradiances  S_vec="[ 1000  500  100 ]"  Temp_C_vec="[ 45 25  ]"  ModuleName=User-defined  PlotWhenSelected=off  Pm=3.8061  Ncell=1  Voc=0.7315  Isc=6.41  Vm=0.626  Im=6.08  beta_Voc_pc=-0.2256195755  alpha_Isc_pc=0.04692556634  beta_Voc=-0.0016504  alpha_Isc=0.0030079  IL=6.4137  I0=6.5578e-13  nI=0.95237  Rsh=7.312  Rs=0.0042689  RobustModel=on  RobustCellTemperature=25  BAL=on  Tc=1e-5  Tfilter=5e-5
  Terminator1 : Terminator
  Variable Resistor2 : spsVariableResistorLib/Variable Resistor  Rabsmin=1e-3
      settings: LibrarySourceBlock=sps_lib/Passives/Variable Resistor
  + : PMIOPort  Side=Left
  - : PMIOPort  Port=2  Side=Right
  wires:
  Irr/1 -> PV2/1
  1PΩ/1 -> Variable Resistor2/1
  PV2/1 -> Terminator1/1
  connections:
  -/RConn1 -- Variable Resistor2/RConn1 -- PV2/RConn2
  +/RConn1 -- Variable Resistor2/LConn1 -- PV2/RConn1

== system WSC_2023_Final_PVArray_Diode_All_Strings/Subsystem29/PV1 ==
  Irr : Inport
  1PΩ : Constant  Value=1e15
  PV1 : spsPVArrayLib/PV Array  Npar=1  Nser=1  PlotType=array @ 25 deg.C & specified irradiances  S_vec="[ 1000  500  100 ]"  Temp_C_vec="[ 45 25  ]"  ModuleName=User-defined  PlotWhenSelected=off  Pm=3.8061  Ncell=1  Voc=0.7315  Isc=6.41  Vm=0.626  Im=6.08  beta_Voc_pc=-0.2256195755  alpha_Isc_pc=0.04692556634  beta_Voc=-0.0016504  alpha_Isc=0.0030079  IL=6.4137  I0=6.5578e-13  nI=0.95237  Rsh=7.312  Rs=0.0042689  RobustModel=on  RobustCellTemperature=25  BAL=on  Tc=1e-5  Tfilter=5e-5
  Terminator1 : Terminator
  Variable Resistor2 : spsVariableResistorLib/Variable Resistor  Rabsmin=1e-3
      settings: LibrarySourceBlock=sps_lib/Passives/Variable Resistor
  + : PMIOPort  Side=Left
  - : PMIOPort  Port=2  Side=Right
  wires:
  Irr/1 -> PV1/1
  1PΩ/1 -> Variable Resistor2/1
  PV1/1 -> Terminator1/1
  connections:
  PV1/RConn2 -- -/RConn1 -- Variable Resistor2/RConn1
  +/RConn1 -- Variable Resistor2/LConn1 -- PV1/RConn1

== system WSC_2023_Final_PVArray_Diode_All_Strings/Subsystem29/PV10 ==
  Irr : Inport
  1PΩ : Constant  Value=1e15
  PV1 : spsPVArrayLib/PV Array  Npar=1  Nser=1  PlotType=array @ 25 deg.C & specified irradiances  S_vec="[ 1000  500  100 ]"  Temp_C_vec="[ 45 25  ]"  ModuleName=User-defined  PlotWhenSelected=off  Pm=3.8061  Ncell=1  Voc=0.7315  Isc=6.41  Vm=0.626  Im=6.08  beta_Voc_pc=-0.2256195755  alpha_Isc_pc=0.04692556634  beta_Voc=-0.0016504  alpha_Isc=0.0030079  IL=6.4137  I0=6.5578e-13  nI=0.95237  Rsh=7.312  Rs=0.0042689  RobustModel=on  RobustCellTemperature=25  BAL=on  Tc=1e-5  Tfilter=5e-5
  Terminator1 : Terminator
  Variable Resistor2 : spsVariableResistorLib/Variable Resistor  Rabsmin=1e-3
      settings: LibrarySourceBlock=sps_lib/Passives/Variable Resistor
  + : PMIOPort  Side=Left
  - : PMIOPort  Port=2  Side=Right
  wires:
  Irr/1 -> PV1/1
  1PΩ/1 -> Variable Resistor2/1
  PV1/1 -> Terminator1/1
  connections:
  PV1/RConn2 -- -/RConn1 -- Variable Resistor2/RConn1
  +/RConn1 -- Variable Resistor2/LConn1 -- PV1/RConn1

== system WSC_2023_Final_PVArray_Diode_All_Strings/Subsystem3/PV1 ==
  Irr : Inport
  1PΩ : Constant  Value=1e15
  PV1 : spsPVArrayLib/PV Array  Npar=1  Nser=1  PlotType=array @ 25 deg.C & specified irradiances  S_vec="[ 1000  500  100 ]"  Temp_C_vec="[ 45 25  ]"  ModuleName=User-defined  PlotWhenSelected=off  Pm=3.8061  Ncell=1  Voc=0.7315  Isc=6.41  Vm=0.626  Im=6.08  beta_Voc_pc=-0.2256195755  alpha_Isc_pc=0.04692556634  beta_Voc=-0.0016504  alpha_Isc=0.0030079  IL=6.4137  I0=6.5578e-13  nI=0.95237  Rsh=7.312  Rs=0.0042689  RobustModel=on  RobustCellTemperature=25  BAL=on  Tc=1e-5  Tfilter=5e-5
  Terminator1 : Terminator
  Variable Resistor2 : spsVariableResistorLib/Variable Resistor  Rabsmin=1e-3
      settings: LibrarySourceBlock=sps_lib/Passives/Variable Resistor
  + : PMIOPort  Side=Left
  - : PMIOPort  Port=2  Side=Right
  wires:
  Irr/1 -> PV1/1
  1PΩ/1 -> Variable Resistor2/1
  PV1/1 -> Terminator1/1
  connections:
  PV1/RConn2 -- -/RConn1 -- Variable Resistor2/RConn1
  +/RConn1 -- Variable Resistor2/LConn1 -- PV1/RConn1

== system WSC_2023_Final_PVArray_Diode_All_Strings/Subsystem3/PV10 ==
  Irr : Inport
  1PΩ : Constant  Value=1e15
  PV1 : spsPVArrayLib/PV Array  Npar=1  Nser=1  PlotType=array @ 25 deg.C & specified irradiances  S_vec="[ 1000  500  100 ]"  Temp_C_vec="[ 45 25  ]"  ModuleName=User-defined  PlotWhenSelected=off  Pm=3.8061  Ncell=1  Voc=0.7315  Isc=6.41  Vm=0.626  Im=6.08  beta_Voc_pc=-0.2256195755  alpha_Isc_pc=0.04692556634  beta_Voc=-0.0016504  alpha_Isc=0.0030079  IL=6.4137  I0=6.5578e-13  nI=0.95237  Rsh=7.312  Rs=0.0042689  RobustModel=on  RobustCellTemperature=25  BAL=on  Tc=1e-5  Tfilter=5e-5
  Terminator1 : Terminator
  Variable Resistor2 : spsVariableResistorLib/Variable Resistor  Rabsmin=1e-3
      settings: LibrarySourceBlock=sps_lib/Passives/Variable Resistor
  + : PMIOPort  Side=Left
  - : PMIOPort  Port=2  Side=Right
  wires:
  Irr/1 -> PV1/1
  1PΩ/1 -> Variable Resistor2/1
  PV1/1 -> Terminator1/1
  connections:
  PV1/RConn2 -- -/RConn1 -- Variable Resistor2/RConn1
  +/RConn1 -- Variable Resistor2/LConn1 -- PV1/RConn1

== system WSC_2023_Final_PVArray_Diode_All_Strings/Subsystem30/PV1 ==
  Irr : Inport
  1PΩ : Constant  Value=1e15
  PV1 : spsPVArrayLib/PV Array  Npar=1  Nser=1  PlotType=array @ 25 deg.C & specified irradiances  S_vec="[ 1000  500  100 ]"  Temp_C_vec="[ 45 25  ]"  ModuleName=User-defined  PlotWhenSelected=off  Pm=3.8061  Ncell=1  Voc=0.7315  Isc=6.41  Vm=0.626  Im=6.08  beta_Voc_pc=-0.2256195755  alpha_Isc_pc=0.04692556634  beta_Voc=-0.0016504  alpha_Isc=0.0030079  IL=6.4137  I0=6.5578e-13  nI=0.95237  Rsh=7.312  Rs=0.0042689  RobustModel=on  RobustCellTemperature=25  BAL=on  Tc=1e-5  Tfilter=5e-5
  Terminator1 : Terminator
  Variable Resistor2 : spsVariableResistorLib/Variable Resistor  Rabsmin=1e-3
      settings: LibrarySourceBlock=sps_lib/Passives/Variable Resistor
  + : PMIOPort  Side=Left
  - : PMIOPort  Port=2  Side=Right
  wires:
  Irr/1 -> PV1/1
  1PΩ/1 -> Variable Resistor2/1
  PV1/1 -> Terminator1/1
  connections:
  PV1/RConn2 -- -/RConn1 -- Variable Resistor2/RConn1
  +/RConn1 -- Variable Resistor2/LConn1 -- PV1/RConn1

== system WSC_2023_Final_PVArray_Diode_All_Strings/Subsystem30/PV10 ==
  Irr : Inport
  1PΩ : Constant  Value=1e15
  PV1 : spsPVArrayLib/PV Array  Npar=1  Nser=1  PlotType=array @ 25 deg.C & specified irradiances  S_vec="[ 1000  500  100 ]"  Temp_C_vec="[ 45 25  ]"  ModuleName=User-defined  PlotWhenSelected=off  Pm=3.8061  Ncell=1  Voc=0.7315  Isc=6.41  Vm=0.626  Im=6.08  beta_Voc_pc=-0.2256195755  alpha_Isc_pc=0.04692556634  beta_Voc=-0.0016504  alpha_Isc=0.0030079  IL=6.4137  I0=6.5578e-13  nI=0.95237  Rsh=7.312  Rs=0.0042689  RobustModel=on  RobustCellTemperature=25  BAL=on  Tc=1e-5  Tfilter=5e-5
  Terminator1 : Terminator
  Variable Resistor2 : spsVariableResistorLib/Variable Resistor  Rabsmin=1e-3
      settings: LibrarySourceBlock=sps_lib/Passives/Variable Resistor
  + : PMIOPort  Side=Left
  - : PMIOPort  Port=2  Side=Right
  wires:
  Irr/1 -> PV1/1
  1PΩ/1 -> Variable Resistor2/1
  PV1/1 -> Terminator1/1
  connections:
  PV1/RConn2 -- -/RConn1 -- Variable Resistor2/RConn1
  +/RConn1 -- Variable Resistor2/LConn1 -- PV1/RConn1

== system WSC_2023_Final_PVArray_Diode_All_Strings/Subsystem31/PV1 ==
  Irr : Inport
  1PΩ : Constant  Value=1e15
  PV1 : spsPVArrayLib/PV Array  Npar=1  Nser=1  PlotType=array @ 25 deg.C & specified irradiances  S_vec="[ 1000  500  100 ]"  Temp_C_vec="[ 45 25  ]"  ModuleName=User-defined  PlotWhenSelected=off  Pm=3.8061  Ncell=1  Voc=0.7315  Isc=6.41  Vm=0.626  Im=6.08  beta_Voc_pc=-0.2256195755  alpha_Isc_pc=0.04692556634  beta_Voc=-0.0016504  alpha_Isc=0.0030079  IL=6.4137  I0=6.5578e-13  nI=0.95237  Rsh=7.312  Rs=0.0042689  RobustModel=on  RobustCellTemperature=25  BAL=on  Tc=1e-5  Tfilter=5e-5
  Terminator1 : Terminator
  Variable Resistor2 : spsVariableResistorLib/Variable Resistor  Rabsmin=1e-3
      settings: LibrarySourceBlock=sps_lib/Passives/Variable Resistor
  + : PMIOPort  Side=Left
  - : PMIOPort  Port=2  Side=Right
  wires:
  Irr/1 -> PV1/1
  1PΩ/1 -> Variable Resistor2/1
  PV1/1 -> Terminator1/1
  connections:
  PV1/RConn2 -- -/RConn1 -- Variable Resistor2/RConn1
  +/RConn1 -- Variable Resistor2/LConn1 -- PV1/RConn1

== system WSC_2023_Final_PVArray_Diode_All_Strings/Subsystem31/PV10 ==
  Irr : Inport
  1PΩ : Constant  Value=1e15
  PV1 : spsPVArrayLib/PV Array  Npar=1  Nser=1  PlotType=array @ 25 deg.C & specified irradiances  S_vec="[ 1000  500  100 ]"  Temp_C_vec="[ 45 25  ]"  ModuleName=User-defined  PlotWhenSelected=off  Pm=3.8061  Ncell=1  Voc=0.7315  Isc=6.41  Vm=0.626  Im=6.08  beta_Voc_pc=-0.2256195755  alpha_Isc_pc=0.04692556634  beta_Voc=-0.0016504  alpha_Isc=0.0030079  IL=6.4137  I0=6.5578e-13  nI=0.95237  Rsh=7.312  Rs=0.0042689  RobustModel=on  RobustCellTemperature=25  BAL=on  Tc=1e-5  Tfilter=5e-5
  Terminator1 : Terminator
  Variable Resistor2 : spsVariableResistorLib/Variable Resistor  Rabsmin=1e-3
      settings: LibrarySourceBlock=sps_lib/Passives/Variable Resistor
  + : PMIOPort  Side=Left
  - : PMIOPort  Port=2  Side=Right
  wires:
  Irr/1 -> PV1/1
  1PΩ/1 -> Variable Resistor2/1
  PV1/1 -> Terminator1/1
  connections:
  PV1/RConn2 -- -/RConn1 -- Variable Resistor2/RConn1
  +/RConn1 -- Variable Resistor2/LConn1 -- PV1/RConn1

== system WSC_2023_Final_PVArray_Diode_All_Strings/Subsystem32/PV1 ==
  Irr : Inport
  1PΩ : Constant  Value=1e15
  PV1 : spsPVArrayLib/PV Array  Npar=1  Nser=1  PlotType=array @ 25 deg.C & specified irradiances  S_vec="[ 1000  500  100 ]"  Temp_C_vec="[ 45 25  ]"  ModuleName=User-defined  PlotWhenSelected=off  Pm=3.8061  Ncell=1  Voc=0.7315  Isc=6.41  Vm=0.626  Im=6.08  beta_Voc_pc=-0.2256195755  alpha_Isc_pc=0.04692556634  beta_Voc=-0.0016504  alpha_Isc=0.0030079  IL=6.4137  I0=6.5578e-13  nI=0.95237  Rsh=7.312  Rs=0.0042689  RobustModel=on  RobustCellTemperature=25  BAL=on  Tc=1e-5  Tfilter=5e-5
  Terminator1 : Terminator
  Variable Resistor2 : spsVariableResistorLib/Variable Resistor  Rabsmin=1e-3
      settings: LibrarySourceBlock=sps_lib/Passives/Variable Resistor
  + : PMIOPort  Side=Left
  - : PMIOPort  Port=2  Side=Right
  wires:
  Irr/1 -> PV1/1
  1PΩ/1 -> Variable Resistor2/1
  PV1/1 -> Terminator1/1
  connections:
  PV1/RConn2 -- -/RConn1 -- Variable Resistor2/RConn1
  +/RConn1 -- Variable Resistor2/LConn1 -- PV1/RConn1

== system WSC_2023_Final_PVArray_Diode_All_Strings/Subsystem32/PV10 ==
  Irr : Inport
  1PΩ : Constant  Value=1e15
  PV1 : spsPVArrayLib/PV Array  Npar=1  Nser=1  PlotType=array @ 25 deg.C & specified irradiances  S_vec="[ 1000  500  100 ]"  Temp_C_vec="[ 45 25  ]"  ModuleName=User-defined  PlotWhenSelected=off  Pm=3.8061  Ncell=1  Voc=0.7315  Isc=6.41  Vm=0.626  Im=6.08  beta_Voc_pc=-0.2256195755  alpha_Isc_pc=0.04692556634  beta_Voc=-0.0016504  alpha_Isc=0.0030079  IL=6.4137  I0=6.5578e-13  nI=0.95237  Rsh=7.312  Rs=0.0042689  RobustModel=on  RobustCellTemperature=25  BAL=on  Tc=1e-5  Tfilter=5e-5
  Terminator1 : Terminator
  Variable Resistor2 : spsVariableResistorLib/Variable Resistor  Rabsmin=1e-3
      settings: LibrarySourceBlock=sps_lib/Passives/Variable Resistor
  + : PMIOPort  Side=Left
  - : PMIOPort  Port=2  Side=Right
  wires:
  Irr/1 -> PV1/1
  1PΩ/1 -> Variable Resistor2/1
  PV1/1 -> Terminator1/1
  connections:
  PV1/RConn2 -- -/RConn1 -- Variable Resistor2/RConn1
  +/RConn1 -- Variable Resistor2/LConn1 -- PV1/RConn1

== system WSC_2023_Final_PVArray_Diode_All_Strings/Subsystem33/PV1 ==
  Irr : Inport
  1PΩ : Constant  Value=1e15
  PV1 : spsPVArrayLib/PV Array  Npar=1  Nser=1  PlotType=array @ 25 deg.C & specified irradiances  S_vec="[ 1000  500  100 ]"  Temp_C_vec="[ 45 25  ]"  ModuleName=User-defined  PlotWhenSelected=off  Pm=3.8061  Ncell=1  Voc=0.7315  Isc=6.41  Vm=0.626  Im=6.08  beta_Voc_pc=-0.2256195755  alpha_Isc_pc=0.04692556634  beta_Voc=-0.0016504  alpha_Isc=0.0030079  IL=6.4137  I0=6.5578e-13  nI=0.95237  Rsh=7.312  Rs=0.0042689  RobustModel=on  RobustCellTemperature=25  BAL=on  Tc=1e-5  Tfilter=5e-5
  Terminator1 : Terminator
  Variable Resistor2 : spsVariableResistorLib/Variable Resistor  Rabsmin=1e-3
      settings: LibrarySourceBlock=sps_lib/Passives/Variable Resistor
  + : PMIOPort  Side=Left
  - : PMIOPort  Port=2  Side=Right
  wires:
  Irr/1 -> PV1/1
  1PΩ/1 -> Variable Resistor2/1
  PV1/1 -> Terminator1/1
  connections:
  PV1/RConn2 -- -/RConn1 -- Variable Resistor2/RConn1
  +/RConn1 -- Variable Resistor2/LConn1 -- PV1/RConn1

== system WSC_2023_Final_PVArray_Diode_All_Strings/Subsystem33/PV10 ==
  Irr : Inport
  1PΩ : Constant  Value=1e15
  PV1 : spsPVArrayLib/PV Array  Npar=1  Nser=1  PlotType=array @ 25 deg.C & specified irradiances  S_vec="[ 1000  500  100 ]"  Temp_C_vec="[ 45 25  ]"  ModuleName=User-defined  PlotWhenSelected=off  Pm=3.8061  Ncell=1  Voc=0.7315  Isc=6.41  Vm=0.626  Im=6.08  beta_Voc_pc=-0.2256195755  alpha_Isc_pc=0.04692556634  beta_Voc=-0.0016504  alpha_Isc=0.0030079  IL=6.4137  I0=6.5578e-13  nI=0.95237  Rsh=7.312  Rs=0.0042689  RobustModel=on  RobustCellTemperature=25  BAL=on  Tc=1e-5  Tfilter=5e-5
  Terminator1 : Terminator
  Variable Resistor2 : spsVariableResistorLib/Variable Resistor  Rabsmin=1e-3
      settings: LibrarySourceBlock=sps_lib/Passives/Variable Resistor
  + : PMIOPort  Side=Left
  - : PMIOPort  Port=2  Side=Right
  wires:
  Irr/1 -> PV1/1
  1PΩ/1 -> Variable Resistor2/1
  PV1/1 -> Terminator1/1
  connections:
  PV1/RConn2 -- -/RConn1 -- Variable Resistor2/RConn1
  +/RConn1 -- Variable Resistor2/LConn1 -- PV1/RConn1

== system WSC_2023_Final_PVArray_Diode_All_Strings/Subsystem34/PV1 ==
  Irr : Inport
  1PΩ : Constant  Value=1e15
  PV1 : spsPVArrayLib/PV Array  Npar=1  Nser=1  PlotType=array @ 25 deg.C & specified irradiances  S_vec="[ 1000  500  100 ]"  Temp_C_vec="[ 45 25  ]"  ModuleName=User-defined  PlotWhenSelected=off  Pm=3.8061  Ncell=1  Voc=0.7315  Isc=6.41  Vm=0.626  Im=6.08  beta_Voc_pc=-0.2256195755  alpha_Isc_pc=0.04692556634  beta_Voc=-0.0016504  alpha_Isc=0.0030079  IL=6.4137  I0=6.5578e-13  nI=0.95237  Rsh=7.312  Rs=0.0042689  RobustModel=on  RobustCellTemperature=25  BAL=on  Tc=1e-5  Tfilter=5e-5
  Terminator1 : Terminator
  Variable Resistor2 : spsVariableResistorLib/Variable Resistor  Rabsmin=1e-3
      settings: LibrarySourceBlock=sps_lib/Passives/Variable Resistor
  + : PMIOPort  Side=Left
  - : PMIOPort  Port=2  Side=Right
  wires:
  Irr/1 -> PV1/1
  1PΩ/1 -> Variable Resistor2/1
  PV1/1 -> Terminator1/1
  connections:
  PV1/RConn2 -- -/RConn1 -- Variable Resistor2/RConn1
  +/RConn1 -- Variable Resistor2/LConn1 -- PV1/RConn1
